simulink library "cvs_computer_vision_system_lib"  (R2016b)
settings: Solver=ode45  StartTime=0.0  StopTime=10.0  RelTol=1e-3  EnableMultiTasking=on
values from neighbouring files (symbols this model uses):
  cvs_AR_process_time = round((1/cvs_AR_process_hz)/astrobee_time_step_size)*astrobee_time_step_size    [cvs_computer_vision_system_prep.m]
  cvs_handrail_pixel_noise = sqrt((cvs_landmark_max_pixel_error^2)/3)/3    [cvs_computer_vision_system_prep.m]
  cvs_handrail_process_time = round((1/cvs_handrail_process_hz)/astrobee_time_step_size)*astrobee_time_step_size    [cvs_computer_vision_system_prep.m]
  cvs_landmark_pixel_noise = sqrt((cvs_landmark_max_pixel_error^2)/3)/3    [cvs_computer_vision_system_prep.m]
  cvs_landmark_process_time = round((1/cvs_landmark_process_hz)/astrobee_time_step_size)*astrobee_time_step_size    [cvs_computer_vision_system_prep.m]
  cvs_noise_seed = 123    [cvs_computer_vision_system_init.m]
  cvs_optflow_pixel_noise = sqrt((cvs_optflow_max_pixel_error^2)/3)/3    [cvs_computer_vision_system_prep.m]
undefined symbols (not defined in the file or in its folder): ase_local_mode_docking, ase_local_mode_perching, astrobee_time_step_size, cvs_step_time
undefined symbols (not defined in the file): cvs_cam_max_dist, cvs_cam_min_dist, cvs_cam_num_pixels, cvs_cam_pointing, cvs_navcam_P_B_B_error, cvs_navcam_Q_camIdeal2camTrue_error, cvs_optflow_ids, cvs_optflow_map_error, cvs_optflow_map_iss, cvs_optflow_num_hist, cvs_optflow_num_out, cvs_optflow_process_time, cvs_optflow_valid_mask, cvs_optflow_valid_times, tun_abp_p_navcam_body_body, tun_abp_q_body2navcam, tun_cvs_noise_on, tun_cvs_vocam_focal_length, tun_cvs_vocam_pixel_width
libraries: simulink x6, cvs_computer_vision_system_lib x4, math_utils x3
settings Model: Creator=rhnakamu  LastModifiedBy=jfusco1
settings DataIOCC: LimitDataPoints=on  SaveFormat=Array
settings OptimizationCC: LifeSpan=inf
settings DebuggingCC: AllowSymbolicDim=off  SFUnexpectedBacktrackingDiag=warning  SFNoUnconditionalDefaultTransitionDiag=warning  SFExecutionAtInitializationDiag=none
settings HardwareCC: ProdBitPerPointer=32  ProdBitPerSizeT=32  ProdBitPerPtrDiffT=32  ProdLargestAtomicFloat=None  ProdIntDivRoundTo=Undefined  ProdEndianess=Unspecified  ProdWordSize=32  ProdHWDeviceType=32-bit Generic
settings ModelReferenceCC: PropagateSignalLabelsOutOfModel=off
settings GRTTargetCC: TargetLangStandard=C89/C90 (ANSI)  GeneratePreprocessorConditionals=Disable all
settings ConfigComp: CovMetricSettings=dw  CovHtmlReporting=on  CovSaveCumulativeToWorkspaceVar=on  CovSaveSingleToWorkspaceVar=on  CovExternalEMLEnable=off

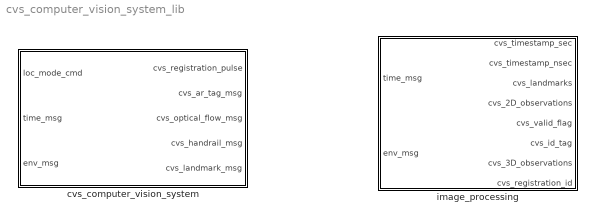
== system cvs_computer_vision_system_lib ==
  cvs_computer_vision_system : Subsystem
  image_processing : Subsystem  mask{system_time=astrobee_time_step_size, process_type=3, process_time=cvs_optflow_process_time, num_points_out=cvs_optflow_num_out, P_point_iss_iss=cvs_optflow_map_iss, valid_flag_mask=cvs_optflow_valid_mask, valid_flag_times=cvs_optflow_valid_times, num_hist_kept=cvs_optflow_num_hist, flow_IDs=cvs_optflow_ids, handrail_vec=0, noise_on_flag=tun_cvs_noise_on, map_error=cvs_optflow_map_error, pixel_noise_seed=cvs_noise_seed*5, pixel_noise_var=cvs_optflow_pixel_noise^2, handrail_noise_var=0, handrail_noise_seed=0, P_cam_B_B=tun_abp_p_navcam_body_body, P_cam_B_B_error=cvs_navcam_P_B_B_error, Q_B2cam=tun_abp_q_body2navcam, Q_B2cam_error=cvs_navcam_Q_camIdeal2camTrue_error, cam_num_X_pixels=cvs_cam_num_pixels(1), cam_num_Y_pixels=cvs_cam_num_pixels(2), cam_focal_length_X=tun_cvs_vocam_focal_length, cam_focal_length_Y=tun_cvs_vocam_pixel_width, cam_pointing=cvs_cam_pointing, cam_min_dist=cvs_cam_min_dist, cam_max_dist=cvs_cam_max_dist}
      mask prompts: system_time "System Time (step time)"; process_type "(1: Landmark, 2: AR Tag, 3: Optical Flow, 4: Handrail)"; process_time "Sample Time (image processing time)"; num_points_out "Number of Points in Output"; P_point_iss_iss "Map Point Positions (P_point_iss_iss)"; valid_flag_mask "Valid Flag Mask"; valid_flag_times "Valid Flag Mask Times"; num_hist_kept "Number of Histories Kept (optical flow only)"; flow_IDs "Map ID values (optical flow only)"; handrail_vec "Handrail Vector (handrail only)"; noise_on_flag "Noise On Flag"; map_error "Map Error"; pixel_noise_seed "Pixel Noise Seed"; pixel_noise_var "Pixel Noise Variance"; handrail_noise_var "Handrail Output Noise Variance"; handrail_noise_seed "Handrail Noise Seed"; P_cam_B_B "Camera Position Nominal (P_cam_B_B)"; P_cam_B_B_error "Camera Position Error"; Q_B2cam "Camera Orientation Nominal (Q_B2cam)"; Q_B2cam_error "Camera Orientation Error"; cam_num_X_pixels "Number of X Pixels"; cam_num_Y_pixels "Number of Y Pixels"; cam_focal_length_X "Image Focal Length X"; cam_focal_length_Y "Image Focal Length Y"; cam_pointing "Lens Pointing Vector (in camera frame)"; cam_min_dist "Minimum Viewing Distance"; cam_max_dist "Maximum Viewing Distance"
      settings: AttributesFormatString=See Mask For Parameter Values
      mask DialogControl DescGroupVar Prompt: Camera Model
      mask DialogControl DescTextVar Prompt: A generic model using pinhole projection

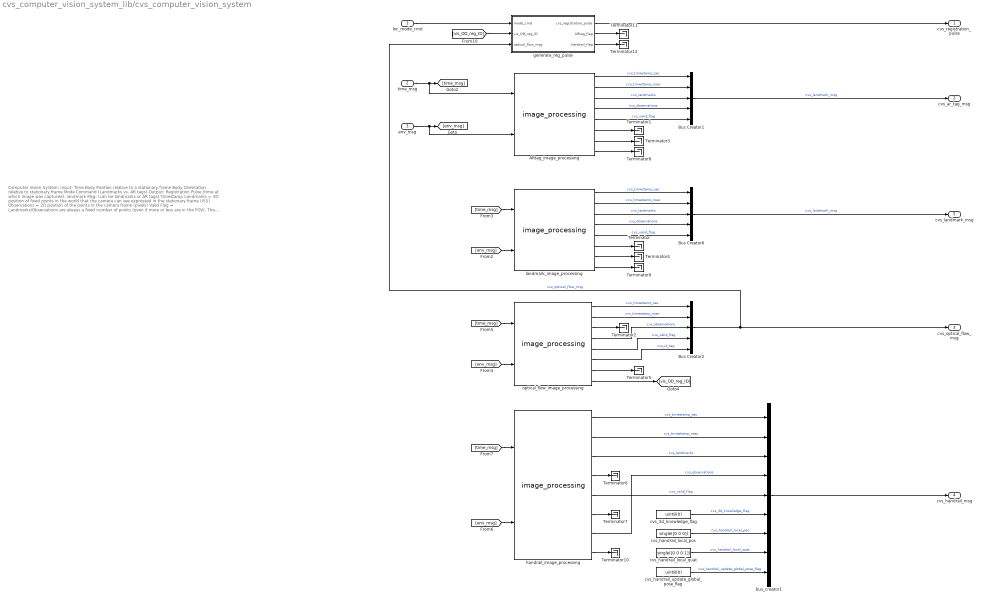
== system cvs_computer_vision_system_lib/cvs_computer_vision_system ==
  note: Computer Vision System:
      | Input:
      | Time
      | Body Position relative to a stationary frame
      | Body Orientation relative to stationary frame
      | Mode Command (Landmarks vs. AR tags)
      | Output:
      | Registration Pulse (time at which image was captured).
      | landmark Msg: (can be landmarks or AR tags)
      | Timestamp
      | Landmarks = 3D position of fixed points in the world that the camera can see expressed in the stationary frame (ISS)
      | Observations = 2D position of the points in the camera frame (pixels)
      | Valid Flag = Landmarks/Observations are always a fixed number of points (even if more or less are in the FOV). This flag indicates 1 if the cooresponding point is valid, 0 if not.
      | optical flow msg:
      | Timestamp
      | observations = 2D position of the points in the camera frame (pixels) for the past N images
      | valid Flag = since observations are always a fixed size, this indicates which are valid
      | Notes:
      | 1) "points" refer to the fixed world points. These are specified in the constant defined in the init file.
      | 2) The general idea here is that a registration pulse is sent at the time a landmark image is captured. This image is then processed for a certain amount of time
      | and then sent out in the message. Immediately after this, another image is captured (sending out another registration pulse).
      | 3) Assumes a rectangular field of view, with square pixels. This assumption is handled in the init/prep files by determining the pixel width/height and # of pixels
  loc_mode_cmd : Inport
  time_msg : Inport  Port=2
  env_msg : Inport  Port=3
  ARtag_image_processing : cvs_computer_vision_system_lib/image_processing  system_time=astrobee_time_step_size  process_type=2  process_time=cvs_AR_process_time  num_points_out=cvs_AR_num_out  P_point_iss_iss=cvs_AR_map_iss  valid_flag_mask=cvs_AR_valid_mask  valid_flag_times=cvs_AR_valid_times  num_hist_kept=0  flow_IDs=0  handrail_vec=0  noise_on_flag=tun_cvs_noise_on  map_error=cvs_AR_map_error  pixel_noise_seed=cvs_noise_seed*4  pixel_noise_var=cvs_AR_pixel_noise  handrail_noise_var=0  handrail_noise_seed=0  P_cam_B_B=tun_abp_p_dockcam_body_body_sim  P_cam_B_B_error=cvs_dockcam_P_B_B_error  Q_B2cam=tun_abp_q_body2dockcam  Q_B2cam_error=cvs_dockcam_Q_B2dockcam_error  cam_num_X_pixels=tun_cvs_dockcam_num_pixels_X  cam_num_Y_pixels=tun_cvs_dockcam_num_pixels_Y  cam_focal_length_X=tun_cvs_dockcam_focal_length_X  cam_focal_length_Y=tun_cvs_dockcam_focal_length_Y  cam_pointing=cvs_dockcam_pointing  cam_min_dist=cvs_dockcam_min_dist  cam_max_dist=cvs_dockcam_max_dist
      settings: AttributesFormatString=See Mask For Parameter Values
  Bus Creator1 : BusCreator  Inputs=5  OutDataTypeStr=Bus: cvs_landmark_msg  NonVirtualBus=on
      settings: InheritFromInputs=off
  Bus Creator2 : BusCreator  Inputs=5  OutDataTypeStr=Bus: cvs_optical_flow_msg  NonVirtualBus=on
      settings: InheritFromInputs=off
  Bus Creator6 : BusCreator  Inputs=5  OutDataTypeStr=Bus: cvs_landmark_msg  NonVirtualBus=on
      settings: InheritFromInputs=off
  Terminator{,1..12} (13 alike) : Terminator
  bus_creator1 : BusCreator  Inputs=9  OutDataTypeStr=Bus: cvs_handrail_msg  NonVirtualBus=on
      settings: InheritFromInputs=off
  cvs_3d_knowledge_flag : Constant  Value=uint8(0)
  cvs_handrail_local_pos : Constant  Value=single([0 0 0])
  cvs_handrail_local_quat : Constant  Value=single([0 0 0 1])
  cvs_handrail_update_global_pose_flag : Constant  Value=uint8(0)
  generate_reg_pulse : Subsystem
  handrail_image_processing : cvs_computer_vision_system_lib/image_processing  system_time=astrobee_time_step_size  process_type=4  process_time=cvs_handrail_process_time  num_points_out=cvs_handrail_num_out  P_point_iss_iss=cvs_handrail_map_iss  valid_flag_mask=cvs_handrail_valid_mask  valid_flag_times=cvs_handrail_valid_times  num_hist_kept=0  flow_IDs=0  handrail_vec=cvs_handrail_vector  noise_on_flag=tun_cvs_noise_on  map_error=cvs_handrail_map_error  pixel_noise_seed=cvs_noise_seed*7  pixel_noise_var=cvs_handrail_pixel_noise^2  handrail_noise_var=cvs_handrail_noise_var  handrail_noise_seed=cvs_noise_seed*8  P_cam_B_B=tun_abp_p_perchcam_body_body_sim  P_cam_B_B_error=cvs_perchcam_P_B_B_error  Q_B2cam=tun_abp_q_body2perchcam  Q_B2cam_error=cvs_perchcam_Q_B2perchcam_error  cam_num_X_pixels=tun_cvs_perchcam_num_pixels_X  cam_num_Y_pixels=tun_cvs_perchcam_num_pixels_Y  cam_focal_length_X=tun_cvs_perchcam_focal_length_X  cam_focal_length_Y=tun_cvs_perchcam_focal_length_Y  cam_pointing=cvs_perchcam_pointing  cam_min_dist=cvs_perchcam_min_dist  cam_max_dist=cvs_perchcam_max_dist
      settings: AttributesFormatString=See Mask For Parameter Values
  landmark_image_processing : cvs_computer_vision_system_lib/image_processing  system_time=astrobee_time_step_size  process_type=1  process_time=cvs_landmark_process_time  num_points_out=cvs_landmark_num_out  P_point_iss_iss=cvs_landmark_map_iss  valid_flag_mask=cvs_landmark_valid_mask  valid_flag_times=cvs_landmark_valid_times  num_hist_kept=0  flow_IDs=0  handrail_vec=0  noise_on_flag=tun_cvs_noise_on  map_error=cvs_landmark_map_error  pixel_noise_seed=cvs_noise_seed*3  pixel_noise_var=cvs_landmark_pixel_noise^2  handrail_noise_var=0  handrail_noise_seed=0  P_cam_B_B=tun_abp_p_navcam_body_body_sim  P_cam_B_B_error=cvs_navcam_P_B_B_error  Q_B2cam=tun_abp_q_body2navcam  Q_B2cam_error=cvs_navcam_Q_B2navcan_error  cam_num_X_pixels=tun_cvs_navcam_num_pixels_X  cam_num_Y_pixels=tun_cvs_navcam_num_pixels_Y  cam_focal_length_X=tun_cvs_navcam_focal_length_X  cam_focal_length_Y=tun_cvs_navcam_focal_length_Y  cam_pointing=cvs_navcam_pointing  cam_min_dist=cvs_navcam_min_dist  cam_max_dist=cvs_navcam_max_dist
      settings: AttributesFormatString=See Mask For Parameter Values
  optical_flow_image_processing : cvs_computer_vision_system_lib/image_processing  system_time=astrobee_time_step_size  process_type=3  process_time=cvs_optflow_process_time  num_points_out=cvs_optflow_num_out  P_point_iss_iss=cvs_optflow_map_iss  valid_flag_mask=cvs_optflow_valid_mask  valid_flag_times=cvs_optflow_valid_times  num_hist_kept=cvs_optflow_num_hist  flow_IDs=cvs_optflow_ids  handrail_vec=0  noise_on_flag=tun_cvs_noise_on  map_error=cvs_optflow_map_error  pixel_noise_seed=cvs_noise_seed*5  pixel_noise_var=cvs_optflow_pixel_noise^2  handrail_noise_var=0  handrail_noise_seed=0  P_cam_B_B=tun_abp_p_navcam_body_body_sim  P_cam_B_B_error=cvs_navcam_P_B_B_error  Q_B2cam=tun_abp_q_body2navcam  Q_B2cam_error=cvs_navcam_Q_B2navcan_error  cam_num_X_pixels=tun_cvs_navcam_num_pixels_X  cam_num_Y_pixels=tun_cvs_navcam_num_pixels_Y  cam_focal_length_X=tun_cvs_navcam_focal_length_X  cam_focal_length_Y=tun_cvs_navcam_focal_length_Y  cam_pointing=cvs_navcam_pointing  cam_min_dist=cvs_navcam_min_dist  cam_max_dist=cvs_navcam_max_dist
      settings: AttributesFormatString=See Mask For Parameter Values
  cvs_registration_pulse : Outport
  cvs_ar_tag_msg : Outport  Port=2
  cvs_optical_flow_msg : Outport  Port=3
  cvs_handrail_msg : Outport  Port=4
  cvs_landmark_msg : Outport  Port=5
  wires:
  [vis_OD_reg_ID] -> generate_reg_pulse/2(vis_OD_reg_ID)
  optical_flow_image_processing/8 -> [vis_OD_reg_ID]
  handrail_image_processing/8 -> Terminator10/1
  landmark_image_processing/8 -> Terminator9/1
  ARtag_image_processing/8 -> Terminator8/1
  cvs_3d_knowledge_flag/1 -> bus_creator1/6  "cvs_3d_knowledge_flag"
  bus_creator1/1 -> cvs_handrail_msg/1
  generate_reg_pulse/3(handrail_flag) -> Terminator12/1
  handrail_image_processing/6 -> Terminator7/1
  handrail_image_processing/4 -> Terminator6/1
  handrail_image_processing/7 -> bus_creator1/4  "cvs_observations"
  handrail_image_processing/3 -> bus_creator1/3  "cvs_landmarks"
  handrail_image_processing/5 -> bus_creator1/5  "cvs_valid_flag"
  handrail_image_processing/2 -> bus_creator1/2  "cvs_timestamp_nsec"
  handrail_image_processing/1 -> bus_creator1/1  "cvs_timestamp_sec"
  [env_msg] -> handrail_image_processing/2
  [time_msg] -> handrail_image_processing/1
  optical_flow_image_processing/7 -> Terminator5/1
  landmark_image_processing/7 -> Terminator4/1
  ARtag_image_processing/7 -> Terminator3/1
  optical_flow_image_processing/3 -> Terminator2/1
  optical_flow_image_processing/6 -> Bus Creator2/5  "cvs_id_tag"
  optical_flow_image_processing/5 -> Bus Creator2/4  "cvs_valid_flag"
  optical_flow_image_processing/4 -> Bus Creator2/3  "cvs_observations"
  optical_flow_image_processing/2 -> Bus Creator2/2  "cvs_timestamp_nsec"
  optical_flow_image_processing/1 -> Bus Creator2/1  "cvs_timestamp_sec"
  generate_reg_pulse/2(ARtag_flag) -> Terminator11/1
  ARtag_image_processing/6 -> Terminator1/1
  ARtag_image_processing/3 -> Bus Creator1/3  "cvs_landmarks"
  ARtag_image_processing/1 -> Bus Creator1/1  "cvs_timestamp_sec"
  ARtag_image_processing/4 -> Bus Creator1/4  "cvs_observations"
  ARtag_image_processing/2 -> Bus Creator1/2  "cvs_timestamp_nsec"
  ARtag_image_processing/5 -> Bus Creator1/5  "cvs_valid_flag"
  Bus Creator6/1 -> cvs_landmark_msg/1  "cvs_landmark_msg"
  landmark_image_processing/6 -> Terminator/1
  landmark_image_processing/1 -> Bus Creator6/1  "cvs_timestamp_sec"
  landmark_image_processing/2 -> Bus Creator6/2  "cvs_timestamp_nsec"
  landmark_image_processing/5 -> Bus Creator6/5  "cvs_valid_flag"
  landmark_image_processing/3 -> Bus Creator6/3  "cvs_landmarks"
  landmark_image_processing/4 -> Bus Creator6/4  "cvs_observations"
  [env_msg] -> landmark_image_processing/2
  [time_msg] -> landmark_image_processing/1
  [env_msg] -> optical_flow_image_processing/2
  [time_msg] -> optical_flow_image_processing/1
  time_msg/1 -> [time_msg], ARtag_image_processing/1
  env_msg/1 -> [env_msg], ARtag_image_processing/2
  loc_mode_cmd/1 -> generate_reg_pulse/1(mode_cmd)
  Bus Creator1/1 -> cvs_ar_tag_msg/1  "cvs_landmark_msg"
  generate_reg_pulse/1(cvs_registration_pulse) -> cvs_registration_pulse/1
  Bus Creator2/1 -> generate_reg_pulse/3(optical_flow_msg), cvs_optical_flow_msg/1  "cvs_optical_flow_msg"
  cvs_handrail_local_pos/1 -> bus_creator1/7  "cvs_handrail_local_pos"
  cvs_handrail_local_quat/1 -> bus_creator1/8  "cvs_handrail_local_quat"
  cvs_handrail_update_global_pose_flag/1 -> bus_creator1/9  "cvs_handrail_update_global_pose_flag"

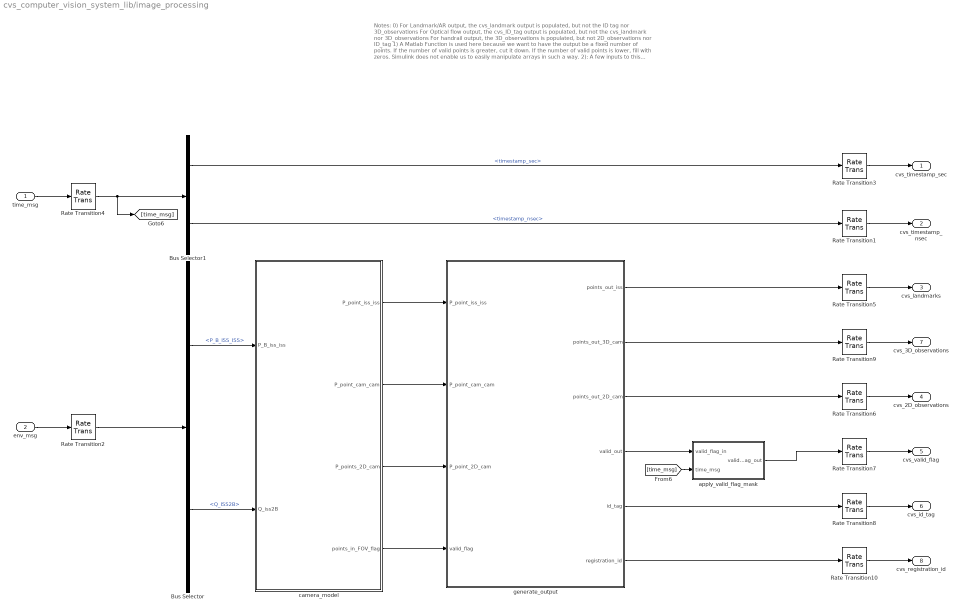
== system cvs_computer_vision_system_lib/image_processing ==
  note: Notes:
      |
      | 0) For Landmark/AR output, the cvs_landmark output is populated, but not the ID tag nor 3D_observations
      | For Optical flow output, the cvs_ID_tag output is populated, but not the cvs_landmark nor 3D_observations
      | For handrail output, the 3D_observations is populated, but not 2D_observations nor ID_tag
      |
      | 1) A Matlab Function is used here because we want to have the output be a fixed number of points.
      | If the number of valid points is greater, cut it down.
      | If the number of valid points is lower, fill with zeros.
      | Simulink does not enable us to easily manipulate arrays in such a way.
      |
      | 2): A few inputs to this function are 'parameterized' since they change the size of the output array
      | To see this, right click the block, then click on 'explore' (library link must be disabled first)
      |
      | 3) The redundant data type conversions enable us to rename the signal
  time_msg : Inport
  env_msg : Inport  Port=2
  Bus Selector : BusSelector  OutputSignals=P_B_ISS_ISS,Q_ISS2B
  Bus Selector1 : BusSelector  OutputSignals=timestamp_sec,timestamp_nsec
  Rate Transition{1,3,5..10} (8 alike) : RateTransition  OutPortSampleTime=system_time
      settings: AttributesFormatString=|
      | IC: %<X0>
      | SampleTime: %<OutPortSampleTime>
  Rate Transition2 : RateTransition  OutPortSampleTime=process_time
      settings: AttributesFormatString=|
      | IC: %<X0>
      | SampleTime: %<OutPortSampleTime>
  Rate Transition4 : RateTransition  OutPortSampleTime=process_time
      settings: AttributesFormatString=|
      | IC: %<X0>
      | SampleTime: %<OutPortSampleTime>
  apply_valid_flag_mask : Subsystem
  camera_model : Subsystem
  generate_output : MATLAB Function  TreatAsAtomicUnit=on
      settings: AttributesFormatString=|
      | Parameter inputs (see notes):
      | process_type
      | num_points_out
      | num_hist_kept
      | flow_ids
  cvs_timestamp_sec : Outport
  cvs_timestamp_nsec : Outport  Port=2
  cvs_landmarks : Outport  Port=3
  cvs_2D_observations : Outport  Port=4
  cvs_valid_flag : Outport  Port=5
  cvs_id_tag : Outport  Port=6
  cvs_3D_observations : Outport  Port=7
  cvs_registration_id : Outport  Port=8
  wires:
  generate_output/6(registration_id) -> Rate Transition10/1
  Rate Transition10/1 -> cvs_registration_id/1
  Rate Transition9/1 -> cvs_3D_observations/1
  generate_output/2(points_out_3D_cam) -> Rate Transition9/1
  camera_model/2(P_point_cam_cam) -> generate_output/2(P_point_cam_cam)
  Rate Transition8/1 -> cvs_id_tag/1
  Rate Transition7/1 -> cvs_valid_flag/1
  Rate Transition6/1 -> cvs_2D_observations/1
  Rate Transition5/1 -> cvs_landmarks/1
  Rate Transition1/1 -> cvs_timestamp_nsec/1
  Rate Transition3/1 -> cvs_timestamp_sec/1
  generate_output/5(id_tag) -> Rate Transition8/1
  generate_output/3(points_out_2D_cam) -> Rate Transition6/1
  generate_output/1(points_out_iss) -> Rate Transition5/1
  camera_model/1(P_point_iss_iss) -> generate_output/1(P_point_iss_iss)
  camera_model/3(P_points_2D_cam) -> generate_output/3(P_point_2D_cam)
  camera_model/4("points_in_FOV_flag ") -> generate_output/4(valid_flag)
  Rate Transition2/1 -> Bus Selector/1
  Rate Transition4/1 -> [time_msg], Bus Selector1/1
  time_msg/1 -> Rate Transition4/1
  env_msg/1 -> Rate Transition2/1
  Bus Selector1/1 -> Rate Transition3/1  "<timestamp_sec>"
  Bus Selector1/2 -> Rate Transition1/1  "<timestamp_nsec>"
  Bus Selector/1 -> camera_model/1(P_B_iss_iss)  "<P_B_ISS_ISS>"
  Bus Selector/2 -> camera_model/2(Q_iss2B)  "<Q_ISS2B>"
  generate_output/4(valid_out) -> apply_valid_flag_mask/1(valid_flag_in)
  apply_valid_flag_mask/1(valid_flag_out) -> Rate Transition7/1
  [time_msg] -> apply_valid_flag_mask/2(time_msg)

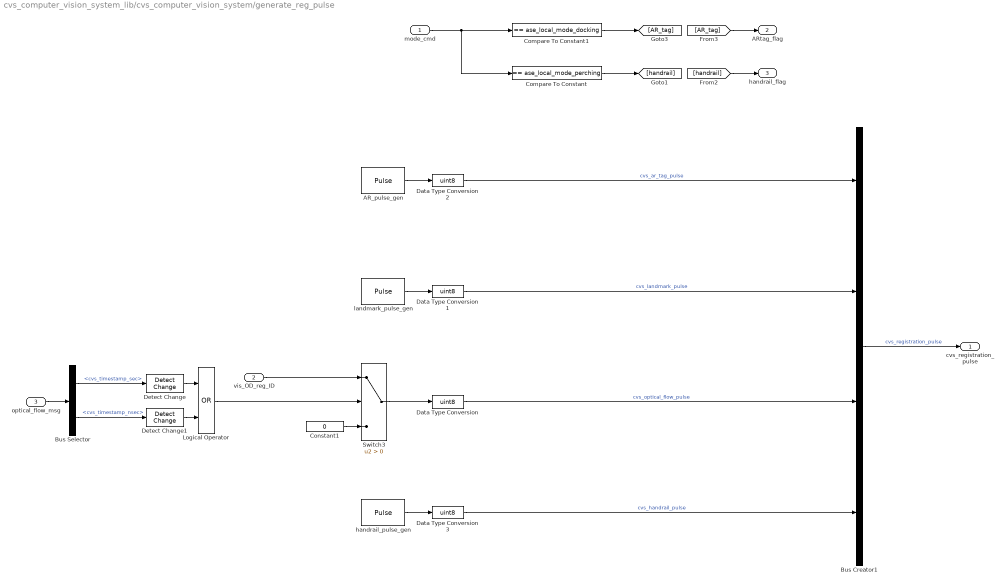
== system cvs_computer_vision_system_lib/cvs_computer_vision_system/generate_reg_pulse ==
  mode_cmd : Inport
  vis_OD_reg_ID : Inport  Port=2
  optical_flow_msg : Inport  Port=3
  AR_pulse_gen : DiscretePulseGenerator  Period=floor(cvs_AR_process_time/astrobee_time_step_size)  SampleTime=astrobee_time_step_size
      settings: AttributesFormatString=|
      | Amp: %<Amplitude>
      | Period: %<Period>
      | Pulse Width: %<PulseWidth>
      | Sample Time: %<SampleTime>
  Bus Creator1 : BusCreator  Inputs=4  OutDataTypeStr=Bus: cvs_registration_pulse  NonVirtualBus=on
      settings: InheritFromInputs=off
  Bus Selector : BusSelector  OutputSignals=cvs_timestamp_sec,cvs_timestamp_nsec
  Compare To Constant : simulink/Logic and Bit Operations/Compare To Constant  relop===  const=ase_local_mode_perching  OutDataTypeStr=boolean
  Compare To Constant1 : simulink/Logic and Bit Operations/Compare To Constant  relop===  const=ase_local_mode_docking  OutDataTypeStr=boolean
  Constant1 : Constant  Value=0
  Data Type Conversion{,1..3} (4 alike) : DataTypeConversion  OutDataTypeStr=uint8
  Detect Change : simulink/Logic and Bit Operations/Detect Change  vinit=0  InputProcessing=Inherited  OutDataTypeStr=boolean
  Detect Change1 : simulink/Logic and Bit Operations/Detect Change  vinit=0  InputProcessing=Inherited  OutDataTypeStr=boolean
  Logical Operator : Logic  Operator=OR  AllPortsSameDT=off  OutDataTypeStr=boolean
  Switch3 : Switch  Criteria=u2 > Threshold
  handrail_pulse_gen : DiscretePulseGenerator  Period=floor(cvs_handrail_process_time/astrobee_time_step_size)  SampleTime=astrobee_time_step_size
      settings: AttributesFormatString=|
      | Amp: %<Amplitude>
      | Period: %<Period>
      | Pulse Width: %<PulseWidth>
      | Sample Time: %<SampleTime>
  landmark_pulse_gen : DiscretePulseGenerator  Period=floor(cvs_landmark_process_time/astrobee_time_step_size)  SampleTime=astrobee_time_step_size
      settings: AttributesFormatString=|
      | Amp: %<Amplitude>
      | Period: %<Period>
      | Pulse Width: %<PulseWidth>
      | Sample Time: %<SampleTime>
  cvs_registration_pulse : Outport
  ARtag_flag : Outport  Port=2
  handrail_flag : Outport  Port=3
  wires:
  Constant1/1 -> Switch3/3
  Logical Operator/1 -> Switch3/2
  vis_OD_reg_ID/1 -> Switch3/1
  Data Type Conversion3/1 -> Bus Creator1/4  "cvs_handrail_pulse"
  handrail_pulse_gen/1 -> Data Type Conversion3/1
  Data Type Conversion1/1 -> Bus Creator1/2  "cvs_landmark_pulse"
  Compare To Constant/1 -> [handrail]
  [handrail] -> handrail_flag/1
  [AR_tag] -> ARtag_flag/1
  Compare To Constant1/1 -> [AR_tag]
  Data Type Conversion/1 -> Bus Creator1/3  "cvs_optical_flow_pulse"
  landmark_pulse_gen/1 -> Data Type Conversion1/1
  Switch3/1 -> Data Type Conversion/1
  Bus Creator1/1 -> cvs_registration_pulse/1  "cvs_registration_pulse"
  mode_cmd/1 -> Compare To Constant/1, Compare To Constant1/1
  AR_pulse_gen/1 -> Data Type Conversion2/1
  Data Type Conversion2/1 -> Bus Creator1/1  "cvs_ar_tag_pulse"
  optical_flow_msg/1 -> Bus Selector/1
  Bus Selector/1 -> Detect Change/1  "<cvs_timestamp_sec>"
  Bus Selector/2 -> Detect Change1/1  "<cvs_timestamp_nsec>"
  Detect Change1/1 -> Logical Operator/2
  Detect Change/1 -> Logical Operator/1

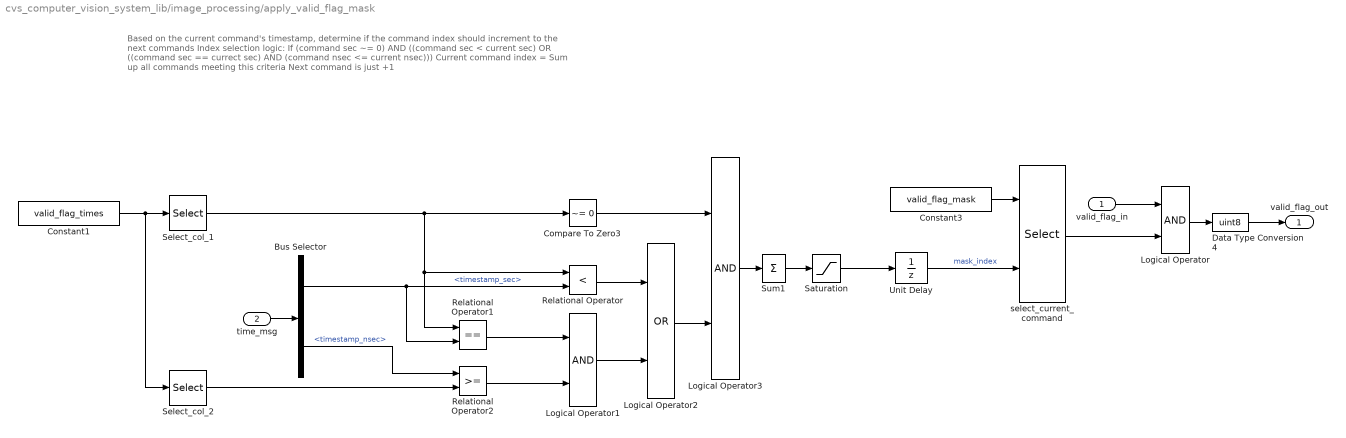
== system cvs_computer_vision_system_lib/image_processing/apply_valid_flag_mask ==
  note: Based on the current command's timestamp, determine if the command index should increment to the next commands
      |
      | Index selection logic:
      | If (command sec ~= 0) AND ((command sec < current sec) OR ((command sec == currect sec) AND (command nsec <= current nsec)))
      | Current command index = Sum up all commands meeting this criteria
      | Next command is just +1
  valid_flag_in : Inport
  time_msg : Inport  Port=2
  Bus Selector : BusSelector  OutputSignals=timestamp_sec,timestamp_nsec
  Compare To Zero3 : simulink/Logic and Bit Operations/Compare To Zero  relop=~=  OutDataTypeStr=boolean
  Constant1 : Constant  Value=valid_flag_times
  Constant3 : Constant  Value=valid_flag_mask
  Data Type Conversion4 : DataTypeConversion  OutDataTypeStr=uint8
  Logical Operator : Logic  AllPortsSameDT=off  OutDataTypeStr=boolean
  Logical Operator1 : Logic  AllPortsSameDT=off  OutDataTypeStr=boolean
  Logical Operator2 : Logic  Operator=OR  AllPortsSameDT=off  OutDataTypeStr=boolean
  Logical Operator3 : Logic  AllPortsSameDT=off  OutDataTypeStr=boolean
  Relational Operator : RelationalOperator  Operator=<  OutDataTypeStr=boolean  RndMeth=Nearest
  Relational Operator1 : RelationalOperator  Operator===  OutDataTypeStr=boolean  RndMeth=Nearest
  Relational Operator2 : RelationalOperator  OutDataTypeStr=boolean  RndMeth=Nearest
  Saturation : Saturate  UpperLimit=length(valid_flag_mask)  LowerLimit=1
      settings: AttributesFormatString=|
      | UL: %<UpperLimit>
      | LL: %<LowerLimit>
  Select_col_1 : Selector  NumberOfDimensions=2  InputPortWidth=3  IndexOptions=Select all,Index vector (dialog)  Indices=[1 3],1  OutputSizes=1,1
  Select_col_2 : Selector  NumberOfDimensions=2  InputPortWidth=3  IndexOptions=Select all,Index vector (dialog)  Indices=[1 3],2  OutputSizes=1,1
  Sum1 : Sum  Inputs=+
  Unit Delay : UnitDelay  InitialCondition=1  SampleTime=-1
      settings: AttributesFormatString=IC: %<InitialCondition>
  select_current_command : Selector  InputPortWidth=length(valid_flag_mask)  IndexOptions=Index vector (port)  Indices=[1 3]  OutputSizes=1
      settings: AttributesFormatString=Input Width: %<InputPortWidth>
  valid_flag_out : Outport
  wires:
  Logical Operator/1 -> Data Type Conversion4/1
  valid_flag_in/1 -> Logical Operator/1
  Data Type Conversion4/1 -> valid_flag_out/1
  Unit Delay/1 -> select_current_command/2  "mask_index"
  Saturation/1 -> Unit Delay/1
  Sum1/1 -> Saturation/1
  Bus Selector/2 -> Relational Operator2/1  "<timestamp_nsec>"
  Bus Selector/1 -> Relational Operator/2, Relational Operator1/2  "<timestamp_sec>"
  Select_col_2/1 -> Relational Operator2/2
  Select_col_1/1 -> Relational Operator1/1, Relational Operator/1, Compare To Zero3/1
  Relational Operator/1 -> Logical Operator2/1
  Logical Operator1/1 -> Logical Operator2/2
  Relational Operator1/1 -> Logical Operator1/1
  Relational Operator2/1 -> Logical Operator1/2
  time_msg/1 -> Bus Selector/1
  Logical Operator3/1 -> Sum1/1
  Compare To Zero3/1 -> Logical Operator3/1
  Logical Operator2/1 -> Logical Operator3/2
  Constant1/1 -> Select_col_2/1, Select_col_1/1
  Constant3/1 -> select_current_command/1
  select_current_command/1 -> Logical Operator/2

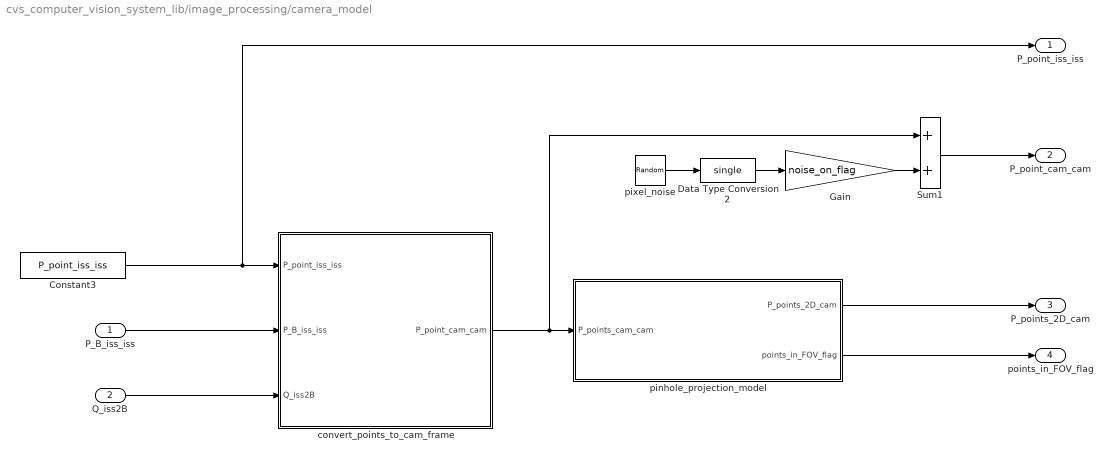
== system cvs_computer_vision_system_lib/image_processing/camera_model ==
  P_B_iss_iss : Inport
  Q_iss2B : Inport  Port=2
  Constant3 : Constant  Value=P_point_iss_iss
  Data Type Conversion2 : DataTypeConversion  OutDataTypeStr=single
  Gain : Gain  Gain=noise_on_flag
  Sum1 : Sum
  convert_points_to_cam_frame : Subsystem  SystemSampleTime=cvs_step_time
  pinhole_projection_model : Subsystem  TreatAsAtomicUnit=on
  pixel_noise : RandomNumber  Variance=handrail_noise_var  Seed=handrail_noise_seed  SampleTime=process_time
      settings: AttributesFormatString=|
      | Variance:%<Variance>
      | Mean:%<Mean>
      | Seed:%<Seed>
      | Sample Time:%<SampleTime>
  P_point_iss_iss : Outport
  P_point_cam_cam : Outport  Port=2
  P_points_2D_cam : Outport  Port=3
  "points_in_FOV_flag " : Outport  Port=4
  wires:
  Q_iss2B/1 -> convert_points_to_cam_frame/3(Q_iss2B)
  pinhole_projection_model/1(P_points_2D_cam) -> P_points_2D_cam/1
  P_B_iss_iss/1 -> convert_points_to_cam_frame/2(P_B_iss_iss)
  convert_points_to_cam_frame/1(P_point_cam_cam) -> Sum1/1, pinhole_projection_model/1(P_points_cam_cam)
  Constant3/1 -> P_point_iss_iss/1, convert_points_to_cam_frame/1(P_point_iss_iss)
  pinhole_projection_model/2(points_in_FOV_flag) -> "points_in_FOV_flag "/1
  Data Type Conversion2/1 -> Gain/1
  pixel_noise/1 -> Data Type Conversion2/1
  Gain/1 -> Sum1/2
  Sum1/1 -> P_point_cam_cam/1

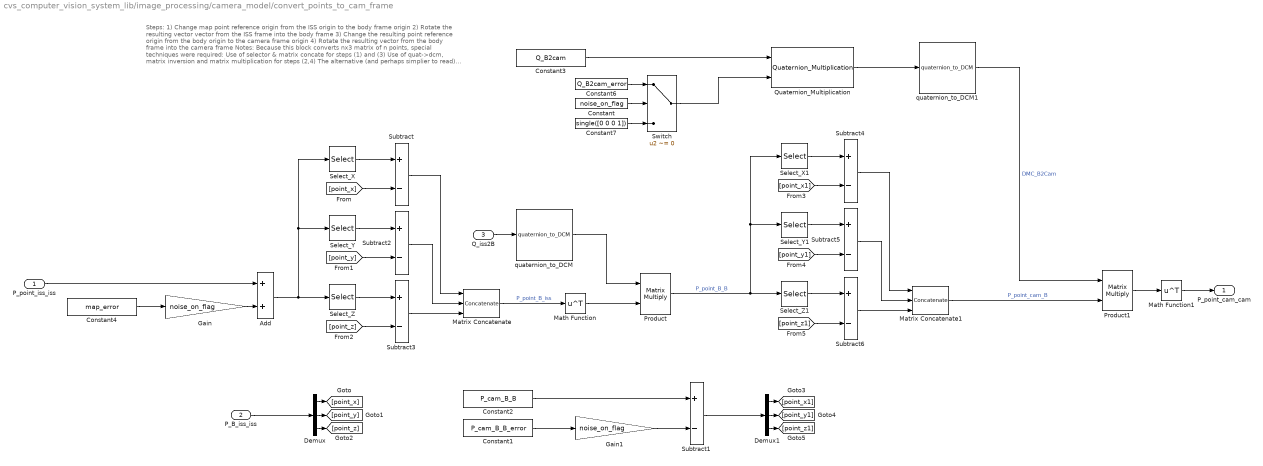
== system cvs_computer_vision_system_lib/image_processing/camera_model/convert_points_to_cam_frame ==
  note: Steps:
      | 	1) Change map point reference origin from the ISS origin to the body frame origin
      | 	2) Rotate the resulting vector vector from the ISS frame into the body frame
      | 	3) Change the resulting point reference origin from the body origin to the camera frame origin
      | 	4) Rotate the resulting vector from the body frame into the camera frame
      |
      | Notes:
      | 	Because this block converts nx3 matrix of n points, special techniques were required:
      | 		Use of selector & matrix concate for steps (1) and (3)
      | 		Use of quat->dcm, matrix inversion and matrix multiplication for steps (2,4)
      | 	The alternative (and perhaps simplier to read) would be to use a "for each" block instead.
  P_point_iss_iss : Inport
  P_B_iss_iss : Inport  Port=2
  Q_iss2B : Inport  Port=3
  Add : Sum
  Constant : Constant  Value=noise_on_flag
  Constant1 : Constant  Value=P_cam_B_B_error
  Constant2 : Constant  Value=P_cam_B_B
  Constant3 : Constant  Value=Q_B2cam
  Constant4 : Constant  Value=map_error
  Constant6 : Constant  Value=Q_B2cam_error
  Constant7 : Constant  Value=single([0 0 0 1])
  Demux : Demux  Outputs=3
  Demux1 : Demux  Outputs=3
  Gain : Gain  Gain=noise_on_flag
  Gain1 : Gain  Gain=noise_on_flag
  Math Function : Math  Operator=transpose  SaturateOnIntegerOverflow=on
  Math Function1 : Math  Operator=transpose  SaturateOnIntegerOverflow=on
  Matrix Concatenate : Concatenate  NumInputs=3  Mode=Multidimensional array  ConcatenateDimension=2
  Matrix Concatenate1 : Concatenate  NumInputs=3  Mode=Multidimensional array
  Product : Product  Multiplication=Matrix(*)
  Product1 : Product  Multiplication=Matrix(*)
  Quaternion_Multiplication : math_utils/Quaternion_Multiplication  SystemSampleTime=-1
  Select_X : Selector  NumberOfDimensions=2  InputPortWidth=3  IndexOptions=Select all,Index vector (dialog)  Indices=[1 3],1  OutputSizes=1,1
  Select_X1 : Selector  NumberOfDimensions=2  InputPortWidth=3  IndexOptions=Index vector (dialog),Select all  Indices=1,1  OutputSizes=1,1
  Select_Y : Selector  NumberOfDimensions=2  InputPortWidth=3  IndexOptions=Select all,Index vector (dialog)  Indices=[1 3],2  OutputSizes=1,1
  Select_Y1 : Selector  NumberOfDimensions=2  InputPortWidth=3  IndexOptions=Index vector (dialog),Select all  Indices=2,2  OutputSizes=1,1
  Select_Z : Selector  NumberOfDimensions=2  InputPortWidth=3  IndexOptions=Select all,Index vector (dialog)  Indices=[1 3],3  OutputSizes=1,1
  Select_Z1 : Selector  NumberOfDimensions=2  InputPortWidth=3  IndexOptions=Index vector (dialog),Select all  Indices=3,3  OutputSizes=1,1
  Subtract{,1..6} (7 alike) : Sum  Inputs=+-
  Switch : Switch  Criteria=u2 ~= 0
  quaternion_to_DCM : math_utils/quaternion_to_DCM  SystemSampleTime=-1
  quaternion_to_DCM1 : math_utils/quaternion_to_DCM  SystemSampleTime=-1
  P_point_cam_cam : Outport
  wires:
  Math Function1/1 -> P_point_cam_cam/1
  Math Function/1 -> Product/2
  quaternion_to_DCM1/1 -> Product1/1  "DMC_B2Cam"
  quaternion_to_DCM/1 -> Product/1
  Subtract6/1 -> Matrix Concatenate1/3
  Subtract5/1 -> Matrix Concatenate1/2
  Subtract4/1 -> Matrix Concatenate1/1
  Demux1/3 -> [point_z1]
  Demux1/2 -> [point_y1]
  Demux1/1 -> [point_x1]
  Select_Z1/1 -> Subtract6/1
  [point_z1] -> Subtract6/2
  [point_y1] -> Subtract5/2
  Select_Y1/1 -> Subtract5/1
  [point_x1] -> Subtract4/2
  Select_X1/1 -> Subtract4/1
  Subtract1/1 -> Demux1/1
  Product/1 -> Select_Z1/1, Select_X1/1, Select_Y1/1  "P_point_B_B"
  Subtract3/1 -> Matrix Concatenate/3
  Subtract2/1 -> Matrix Concatenate/2
  Subtract/1 -> Matrix Concatenate/1
  Demux/3 -> [point_z]
  Demux/2 -> [point_y]
  Demux/1 -> [point_x]
  Select_Z/1 -> Subtract3/1
  [point_z] -> Subtract3/2
  [point_y] -> Subtract2/2
  Select_Y/1 -> Subtract2/1
  [point_x] -> Subtract/2
  Select_X/1 -> Subtract/1
  Product1/1 -> Math Function1/1
  P_B_iss_iss/1 -> Demux/1
  Q_iss2B/1 -> quaternion_to_DCM/1
  Matrix Concatenate/1 -> Math Function/1  "P_point_B_iss"
  Matrix Concatenate1/1 -> Product1/2  "P_point_cam_B"
  Add/1 -> Select_X/1, Select_Y/1, Select_Z/1
  Gain/1 -> Add/2
  Constant4/1 -> Gain/1
  P_point_iss_iss/1 -> Add/1
  Constant2/1 -> Subtract1/1
  Constant1/1 -> Gain1/1
  Gain1/1 -> Subtract1/2
  Switch/1 -> Quaternion_Multiplication/2
  Constant3/1 -> Quaternion_Multiplication/1
  Quaternion_Multiplication/1 -> quaternion_to_DCM1/1
  Constant/1 -> Switch/2
  Constant6/1 -> Switch/1
  Constant7/1 -> Switch/3

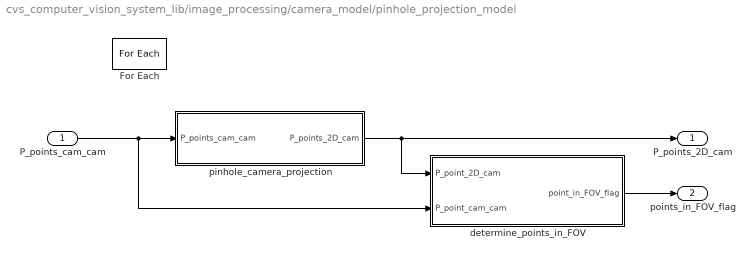
== system cvs_computer_vision_system_lib/image_processing/camera_model/pinhole_projection_model ==
  P_points_cam_cam : Inport  Partition=on  PartitionDimension=1  PartitionWidth=1
  For Each : ForEach  DisableCoverage=on  IndexMode=One-based
  determine_points_in_FOV : Subsystem
  pinhole_camera_projection : Subsystem
  P_points_2D_cam : Outport  ConcatenationDimension=1
  points_in_FOV_flag : Outport  Port=2  ConcatenationDimension=1
  wires:
  pinhole_camera_projection/1(P_points_2D_cam) -> determine_points_in_FOV/1(P_point_2D_cam), P_points_2D_cam/1
  P_points_cam_cam/1 -> pinhole_camera_projection/1(P_points_cam_cam), determine_points_in_FOV/2(P_point_cam_cam)
  determine_points_in_FOV/1(point_in_FOV_flag) -> points_in_FOV_flag/1

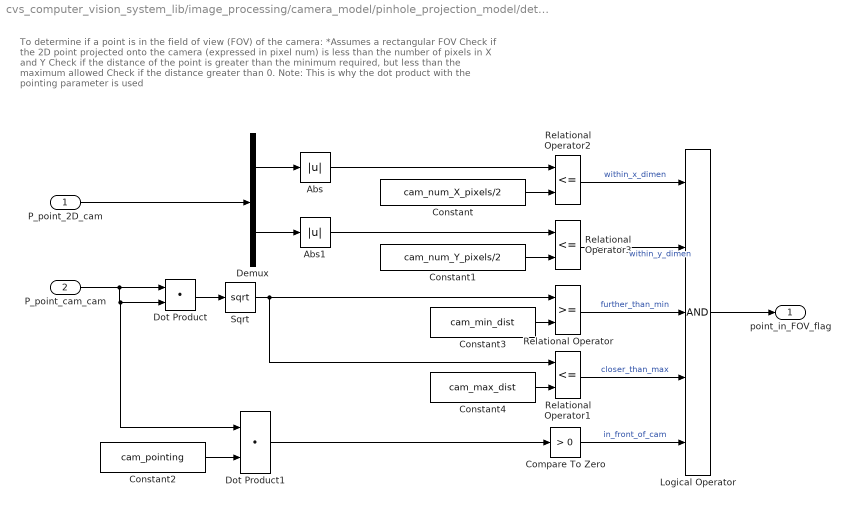
== system cvs_computer_vision_system_lib/image_processing/camera_model/pinhole_projection_model/determine_points_in_FOV ==
  note: To determine if a point is in the field of view (FOV) of the camera:
      | *Assumes a rectangular FOV
      | Check if the 2D point projected onto the camera (expressed in pixel num) is less than the number of pixels in X and Y
      | Check if the distance of the point is greater than the minimum required, but less than the maximum allowed
      | Check if the distance greater than 0. Note: This is why the dot product with the pointing parameter is used
  P_point_2D_cam : Inport
  P_point_cam_cam : Inport  Port=2
  Abs : Abs
  Abs1 : Abs
  Compare To Zero : simulink/Logic and Bit Operations/Compare To Zero  relop=>  OutDataTypeStr=boolean
  Constant : Constant  Value=cam_num_X_pixels/2
  Constant1 : Constant  Value=cam_num_Y_pixels/2
  Constant2 : Constant  Value=cam_pointing
  Constant3 : Constant  Value=cam_min_dist
  Constant4 : Constant  Value=cam_max_dist
  Demux : Demux  Outputs=2
  Dot Product : DotProduct  InputSameDT=on  OutDataTypeStr=Inherit: Inherit via internal rule
  Dot Product1 : DotProduct  InputSameDT=on  OutDataTypeStr=Inherit: Inherit via internal rule
  Logical Operator : Logic  Inputs=5  AllPortsSameDT=off  OutDataTypeStr=boolean
  Relational Operator : RelationalOperator  OutDataTypeStr=boolean  RndMeth=Nearest
  Relational Operator1 : RelationalOperator  Operator=<=  OutDataTypeStr=boolean  RndMeth=Nearest
  Relational Operator2 : RelationalOperator  Operator=<=  OutDataTypeStr=boolean  RndMeth=Nearest
  Relational Operator3 : RelationalOperator  Operator=<=  OutDataTypeStr=boolean  RndMeth=Nearest
  Sqrt : Sqrt  SaturateOnIntegerOverflow=on
  point_in_FOV_flag : Outport
  wires:
  Constant2/1 -> Dot Product1/2
  Compare To Zero/1 -> Logical Operator/5  "in_front_of_cam"
  Dot Product1/1 -> Compare To Zero/1
  Abs1/1 -> Relational Operator3/1
  Abs/1 -> Relational Operator2/1
  Relational Operator2/1 -> Logical Operator/1  "within_x_dimen"
  Relational Operator3/1 -> Logical Operator/2  "within_y_dimen"
  Constant1/1 -> Relational Operator3/2
  Demux/2 -> Abs1/1
  Constant/1 -> Relational Operator2/2
  Demux/1 -> Abs/1
  P_point_2D_cam/1 -> Demux/1
  P_point_cam_cam/1 -> Dot Product/2, Dot Product1/1, Dot Product/1
  Dot Product/1 -> Sqrt/1
  Constant3/1 -> Relational Operator/2
  Constant4/1 -> Relational Operator1/2
  Relational Operator1/1 -> Logical Operator/4  "closer_than_max"
  Relational Operator/1 -> Logical Operator/3  "further_than_min"
  Sqrt/1 -> Relational Operator1/1, Relational Operator/1
  Logical Operator/1 -> point_in_FOV_flag/1

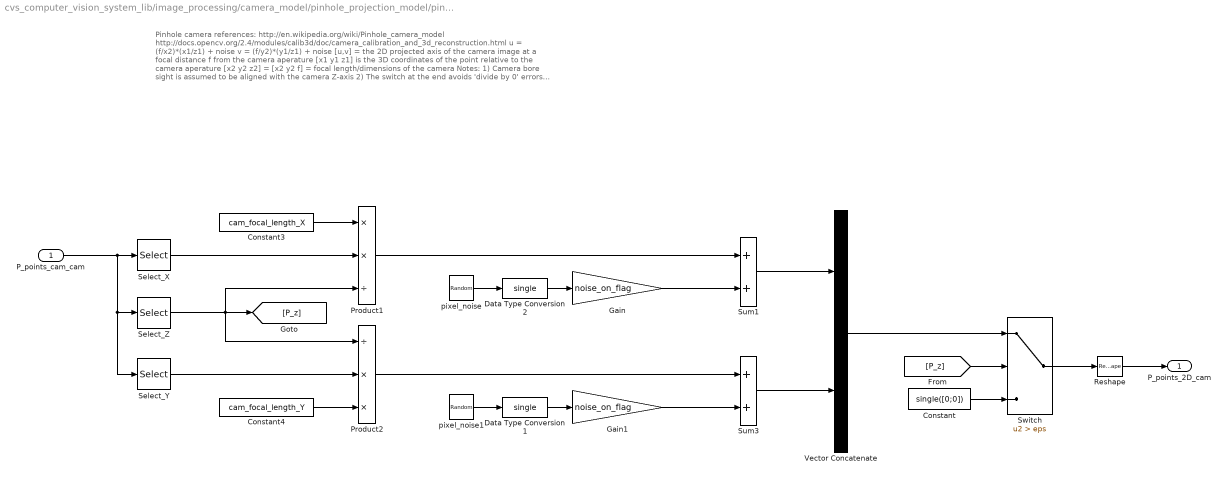
== system cvs_computer_vision_system_lib/image_processing/camera_model/pinhole_projection_model/pinhole_camera_projection ==
  note: Pinhole camera references:
      | http://en.wikipedia.org/wiki/Pinhole_camera_model
      | http://docs.opencv.org/2.4/modules/calib3d/doc/camera_calibration_and_3d_reconstruction.html
      |
      | u = (f/x2)*(x1/z1) + noise
      | v = (f/y2)*(y1/z1) + noise
      | [u,v] = the 2D projected axis of the camera image at a focal distance f from the camera aperature
      | [x1 y1 z1] is the 3D coordinates of the point relative to the camera aperature
      | [x2 y2 z2] = [x2 y2 f] = focal length/dimensions of the camera
      |
      | Notes:
      | 1) Camera bore sight is assumed to be aligned with the camera Z-axis
      | 2) The switch at the end avoids 'divide by 0' errors if the X3 distance to a point is 0.
      | It actually checks if >eps for numerical error reasons. <eps is essentially 0 in matlab
  P_points_cam_cam : Inport
  Constant : Constant  Value=single([0;0])
  Constant3 : Constant  Value=cam_focal_length_X
      settings: AttributesFormatString=|
      | SampleTime: %<SampleTime>
      | Data Type: %<OutDataTypeStr>
  Constant4 : Constant  Value=cam_focal_length_Y
      settings: AttributesFormatString=|
      | SampleTime: %<SampleTime>
      | Data Type: %<OutDataTypeStr>
  Data Type Conversion1 : DataTypeConversion  OutDataTypeStr=single
  Data Type Conversion2 : DataTypeConversion  OutDataTypeStr=single
  Gain : Gain  Gain=noise_on_flag
  Gain1 : Gain  Gain=noise_on_flag
  Product1 : Product  Inputs=**/
  Product2 : Product  Inputs=/**
  Reshape : Reshape  OutputDimensionality=Row vector (2-D)
  Select_X : Selector  InputPortWidth=3  IndexOptions=Index vector (dialog)  Indices=1  OutputSizes=1
  Select_Y : Selector  InputPortWidth=3  IndexOptions=Index vector (dialog)  Indices=2  OutputSizes=1
  Select_Z : Selector  InputPortWidth=3  IndexOptions=Index vector (dialog)  Indices=3  OutputSizes=1
  Sum1 : Sum
  Sum3 : Sum
  Switch : Switch  Criteria=u2 > Threshold  Threshold=eps
      settings: AttributesFormatString=If > %<Threshold>
  Vector Concatenate : Concatenate
  pixel_noise : RandomNumber  Variance=pixel_noise_var  Seed=pixel_noise_seed+1  SampleTime=process_time
      settings: AttributesFormatString=|
      | Variance:%<Variance>
      | Mean:%<Mean>
      | Seed:%<Seed>
      | Sample Time:%<SampleTime>
  pixel_noise1 : RandomNumber  Variance=pixel_noise_var  Seed=pixel_noise_seed+2  SampleTime=process_time
      settings: AttributesFormatString=|
      | Variance:%<Variance>
      | Mean:%<Mean>
      | Seed:%<Seed>
      | Sample Time:%<SampleTime>
  P_points_2D_cam : Outport
  wires:
  Constant4/1 -> Product2/3
  Constant3/1 -> Product1/1
  Data Type Conversion1/1 -> Gain1/1
  Data Type Conversion2/1 -> Gain/1
  [P_z] -> Switch/2
  Constant/1 -> Switch/3
  Select_X/1 -> Product1/2
  Select_Z/1 -> Product2/1, [P_z], Product1/3
  Select_Y/1 -> Product2/2
  P_points_cam_cam/1 -> Select_Z/1, Select_Y/1, Select_X/1
  Switch/1 -> Reshape/1
  Reshape/1 -> P_points_2D_cam/1
  Product2/1 -> Sum3/1
  Vector Concatenate/1 -> Switch/1
  pixel_noise/1 -> Data Type Conversion2/1
  pixel_noise1/1 -> Data Type Conversion1/1
  Sum3/1 -> Vector Concatenate/2
  Sum1/1 -> Vector Concatenate/1
  Gain1/1 -> Sum3/2
  Product1/1 -> Sum1/1
  Gain/1 -> Sum1/2

== matlab function cvs_computer_vision_system_lib/image_processing/generate_output ==
  data: process_type parameter; num_points_out parameter; points_out_iss output; points_out_3D_cam output; points_out_2D_cam output; valid_out output; P_point_iss_iss input; P_point_cam_cam input; P_point_2D_cam input; valid_flag input; id_tag output; num_hist_kept parameter; flow_IDs parameter; registration_id output
function [points_out_iss, points_out_3D_cam, points_out_2D_cam, valid_out, id_tag, registration_id] = generate_output(process_type, num_points_out, P_point_iss_iss, P_point_cam_cam, P_point_2D_cam, valid_flag, num_hist_kept, flow_IDs)
%#codegen

% Inputs:
%   Process type:                                                                [Parameter]
%       1=Landmarks, 2=AR Tags, 3=Optical Flow, 4=Handrail
%   num_pts_out         = Required number of points to be reported               [Parameter]
%   P_point_iss_iss     = ALL [x,y,z] position of points in the ISS frame        **Landmark only**
%   P_point_cam_cam     = ALL [x,y,z] position of points in the CAM frame        **Handrail only**
%   P_points_2D_cam     = ALL [u,v] pixel location of points in the camera       **Landmark and OF only**
%   valid_flag          = indicates which points are valid
%   num_hist_kept       = Required number of histories kept for Optical Flow     [Parameter] **OF only**
%   flow_ids            = ID tag for each optical flow point                     [Parameter] **OF only**
%
% Outputs:
%   points_out_iss      = output [x,y,z] position of points in the ISS frame     **This output unused by optical flow**
%   points_out_2D_cam   = output [u,v] pixel location of points in the camera    **This output unused by handrail**
%   points_out_cam      = output [x,y,z] position of points in the CAM frame     **This output unused by OF and landmarks**
%   valid_out           = indicates which values of the output are valid!        **This output unused by landmarks**
%   ids_out             = optical flow IDs
%   registration_id     = visual odometery registration pulse ID                 **ONLY used by OF**

switch process_type
    case 4  %handrail
        [points_out_iss, points_out_3D_cam, valid_out]  = format_handrail_output(num_points_out, P_point_iss_iss, P_point_cam_cam, valid_flag);
        points_out_2D_cam   = 0;
        id_tag              = 0;
        registration_id     = 1;
    case 3  %optical flow
        [points_out_2D_cam, valid_out, id_tag, registration_id]  = format_optflow_output(num_points_out, P_point_2D_cam, valid_flag, num_hist_kept, flow_IDs);
        points_out_iss      = 0; %landmarks NOT populated/used by optical flow
        points_out_3D_cam   = 0; %cam points not populated by OF
    case 2  %AR tags
        [points_out_iss, points_out_2D_cam, valid_out]  = format_AR_tag_output(num_points_out, P_point_iss_iss, P_point_2D_cam, valid_flag);
        id_tag              = 0;
        points_out_3D_cam   = 0;
        registration_id     = 1;
    otherwise %default to landmarks
        [points_out_iss, points_out_2D_cam, valid_out]  = format_landmark_output(num_points_out, P_point_iss_iss, P_point_2D_cam, valid_flag);
        id_tag              = 0; %ID tag only populated/used in optical flow
        points_out_3D_cam   = 0; %cam points not populated by landmarks
        registration_id     = 1;
end

%end of function
end
